simulink model "tsfinatohardware"  (R2024a)
settings: Solver=VariableStepAuto  StartTime=0.0  StopTime=10.0  RelTol=1e-3
settings Model: Creator=Abhilash LN  LastModifiedBy=Abhilash LN

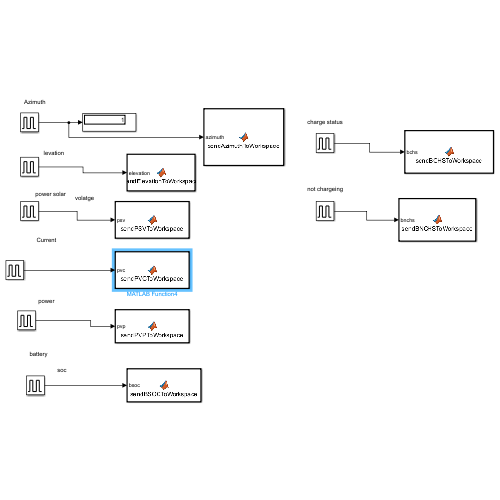
[thumbnail: Simulink's stored preview of the top-level diagram]
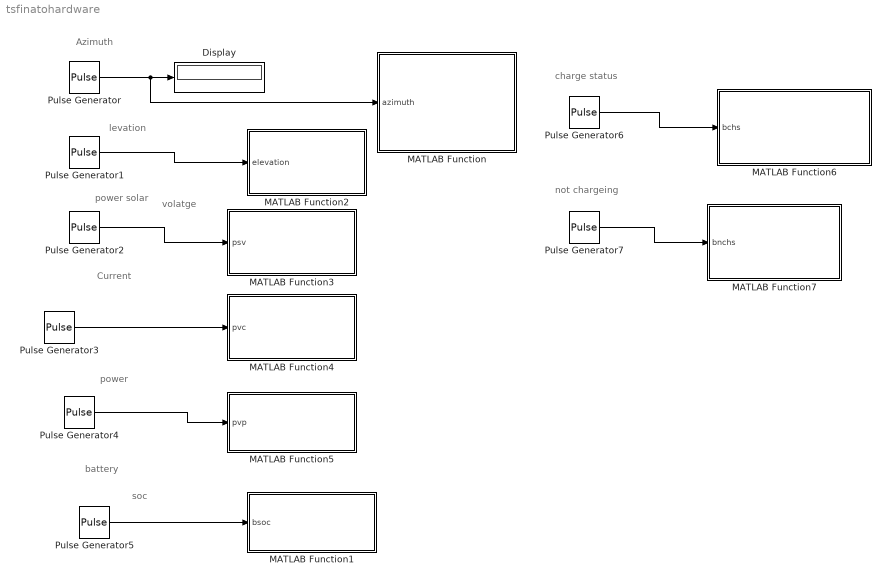
== system tsfinatohardware ==
  note: not chargeing
  note: charge status
  note: soc
  note: battery
  note: power
  note: Current
  note: volatge
  note: power solar
  note: levation
  note: Azimuth
  Display : Display
  MATLAB Function : MATLAB Function  TreatAsAtomicUnit=on
  MATLAB Function1 : MATLAB Function  TreatAsAtomicUnit=on
  MATLAB Function2 : MATLAB Function  TreatAsAtomicUnit=on
  MATLAB Function3 : MATLAB Function  TreatAsAtomicUnit=on
  MATLAB Function4 : MATLAB Function  TreatAsAtomicUnit=on
  MATLAB Function5 : MATLAB Function  TreatAsAtomicUnit=on
  MATLAB Function6 : MATLAB Function  TreatAsAtomicUnit=on
  MATLAB Function7 : MATLAB Function  TreatAsAtomicUnit=on
  Pulse Generator{,1..7} (8 alike) : DiscretePulseGenerator  PulseType=Time based  Period=10  PulseWidth=5
  wires:
  Pulse Generator/1 -> MATLAB Function/1(azimuth), Display/1
  Pulse Generator4/1 -> MATLAB Function5/1(pvp)
  Pulse Generator3/1 -> MATLAB Function4/1(pvc)
  Pulse Generator2/1 -> MATLAB Function3/1(psv)
  Pulse Generator1/1 -> MATLAB Function2/1(elevation)
  Pulse Generator5/1 -> MATLAB Function1/1(bsoc)
  Pulse Generator6/1 -> MATLAB Function6/1(bchs)
  Pulse Generator7/1 -> MATLAB Function7/1(bnchs)

== matlab function tsfinatohardware/MATLAB Function ==
  data: azimuth input
function sendAzimuthToWorkspace(azimuth)
    %#codegen

    % Access the shared variable using the Data Store Memory block
    coder.extrinsic('evalin');
    coder.extrinsic('assignin');
    coder.extrinsic('pause'); % Enable use of the pause function

    % Read the current stored array from the workspace
    tsAzimuth = evalin('base', 'tsAzimuth');

    % Initialize if the variable is empty
    if isempty(tsAzimuth)
        tsAzimuth = []; % Start with an empty array if tsAzimuth doesn't exist
    end

    % Ensure the azimuth value is a scalar (or single value)
    if ~isscalar(azimuth)
        error('azimuth must be a scalar value.');
    end

    % Append the new azimuth value to the array as a new column
    tsAzimuth = [tsAzimuth, azimuth]; % Append azimuth as a new column in the array

    % Add a delay of 10 seconds (optional)
    pause(10);

    % Update the workspace variable with the new array
    assignin('base', 'tsAzimuth', tsAzimuth);
end

== matlab function tsfinatohardware/MATLAB Function2 ==
  data: elevation input
function sendElevationToWorkspace(elevation)
    %#codegen

    % Access the shared variable using the Data Store Memory block
    coder.extrinsic('evalin');
    coder.extrinsic('assignin');
    coder.extrinsic('pause'); % Enable use of the pause function

    % Read the current stored array from the workspace
    tsElevation = evalin('base', 'tsElevation');

    % Initialize if the variable is empty
    if isempty(tsElevation)
        tsElevation = []; % Start with an empty array if tsElevation doesn't exist
    end

    % Ensure the elevation value is a scalar (or single value)
    if ~isscalar(elevation)
        error('elevation must be a scalar value.');
    end

    % Append the new elevation value to the array as a new column
    tsElevation = [tsElevation, elevation]; % Append elevation as a new column in the array

    % Add a delay of 10 seconds (optional)
    pause(10);

    % Update the workspace variable with the new array
    assignin('base', 'tsElevation', tsElevation);
end

== matlab function tsfinatohardware/MATLAB Function3 ==
  data: psv input
function sendPSVToWorkspace(psv)
    %#codegen

    % Access the shared variable using the Data Store Memory block
    coder.extrinsic('evalin');
    coder.extrinsic('assignin');
    coder.extrinsic('pause'); % Enable use of the pause function

    % Read the current stored array from the workspace
    tspsv = evalin('base', 'tspsv');

    % Initialize if the variable is empty
    if isempty(tspsv)
        tspsv = []; % Start with an empty array if tspsv doesn't exist
    end

    % Ensure the psv value is a scalar (or single value)
    if ~isscalar(psv)
        error('psv must be a scalar value.');
    end

    % Append the new psv value to the array as a column
    tspsv = [tspsv, psv]; % Append psv as a new column

    % Add a delay of 10 seconds (optional)
    pause(10);

    % Update the workspace variable with the new array
    assignin('base', 'tspsv', tspsv);
end

== matlab function tsfinatohardware/MATLAB Function4 ==
  data: pvc input
function sendPVCToWorkspace(pvc)
    %#codegen

    % Access the shared variable using the Data Store Memory block
    coder.extrinsic('evalin');
    coder.extrinsic('assignin');
    coder.extrinsic('pause'); % Enable use of the pause function

    % Read the current stored array from the workspace
    tspvc = evalin('base', 'tspvc');

    % Initialize if the variable is empty
    if isempty(tspvc)
        tspvc = []; % Start with an empty array if tspvc doesn't exist
    end

    % Ensure the pvc value is a scalar (or single value)
    if ~isscalar(pvc)
        error('pvc must be a scalar value.');
    end

    % Append the new pvc value to the array as a column
    tspvc = [tspvc, pvc]; % Append pvc as a new column

    % Add a delay of 10 seconds (optional)
    pause(10);

    % Update the workspace variable with the new array
    assignin('base', 'tspvc', tspvc);
end

== matlab function tsfinatohardware/MATLAB Function5 ==
  data: pvp input
function sendPVPToWorkspace(pvp)
    %#codegen

    % Access the shared variable using the Data Store Memory block
    coder.extrinsic('evalin');
    coder.extrinsic('assignin');
    coder.extrinsic('pause'); % Enable use of the pause function

    % Read the current stored array from the workspace
    tspvp = evalin('base', 'tspvp');

    % Initialize if the variable is empty
    if isempty(tspvp)
        tspvp = []; % Start with an empty array if tspvp doesn't exist
    end

    % Ensure the pvp value is a scalar (or single value)
    if ~isscalar(pvp)
        error('pvp must be a scalar value.');
    end

    % Append the new pvp value to the array as a column
    tspvp = [tspvp, pvp]; % Append pvp as a new column

    % Add a delay of 10 seconds (optional)
    pause(10);

    % Update the workspace variable with the new array
    assignin('base', 'tspvp', tspvp);
end

== matlab function tsfinatohardware/MATLAB Function6 ==
  data: bchs input
function sendBCHSToWorkspace(bchs)
    %#codegen

    % Access the shared variable using the Data Store Memory block
    coder.extrinsic('evalin');
    coder.extrinsic('assignin');
    coder.extrinsic('pause'); % Enable use of the pause function

    % Read the current stored array from the workspace
    tsbchs = evalin('base', 'tsbchs');

    % Initialize if the variable is empty
    if isempty(tsbchs)
        tsbchs = []; % Start with an empty array if tsbchs doesn't exist
    end

    % Ensure the bchs value is a scalar (or single value)
    if ~isscalar(bchs)
        error('bchs must be a scalar value.');
    end

    % Append the new bchs value to the array as a column
    tsbchs = [tsbchs, bchs]; % Append bchs as a new column

    % Add a delay of 10 seconds (optional)
    pause(10);

    % Update the workspace variable with the new array
    assignin('base', 'tsbchs', tsbchs);
end

== matlab function tsfinatohardware/MATLAB Function7 ==
  data: bnchs input
function sendBNCHSToWorkspace(bnchs)
    %#codegen

    % Access the shared variable using the Data Store Memory block
    coder.extrinsic('evalin');
    coder.extrinsic('assignin');
    coder.extrinsic('pause'); % Enable use of the pause function

    % Read the current stored array from the workspace
    tsbnchs = evalin('base', 'tsbnchs');

    % Initialize if the variable is empty
    if isempty(tsbnchs)
        tsbnchs = []; % Start with an empty array if tsbnchs doesn't exist
    end

    % Ensure the bnchs value is a scalar (or single value)
    if ~isscalar(bnchs)
        error('bnchs must be a scalar value.');
    end

    % Append the new bnchs value to the array as a column
    tsbnchs = [tsbnchs, bnchs]; % Append bnchs as a new column

    % Add a delay of 10 seconds (optional)
    pause(10);

    % Update the workspace variable with the new array
    assignin('base', 'tsbnchs', tsbnchs);
end

== matlab function tsfinatohardware/MATLAB Function1 ==
  data: bsoc input
function sendBSOCToWorkspace(bsoc)
    %#codegen

    % Access the shared variable using the Data Store Memory block
    coder.extrinsic('evalin');
    coder.extrinsic('assignin');
    coder.extrinsic('pause'); % Enable use of the pause function

    % Read the current stored array from the workspace
    tsbsoc = evalin('base', 'tsbsoc');

    % Initialize if the variable is empty
    if isempty(tsbsoc)
        tsbsoc = []; % Start with an empty array if tsbsoc doesn't exist
    end

    % Ensure the bsoc value is a scalar (or single value)
    if ~isscalar(bsoc)
        error('bsoc must be a scalar value.');
    end

    % Append the new bsoc value to the array as a column
    tsbsoc = [tsbsoc, bsoc]; % Append bsoc as a new column

    % Add a delay of 10 seconds (optional)
    pause(10);

    % Update the workspace variable with the new array
    assignin('base', 'tsbsoc', tsbsoc);
end
